simulink model "reaction_wheel_windup"  (R2021b)
settings: Solver=VariableStepAuto  StartTime=0.0  StopTime=200  RelTol=2.82e-14
values from neighbouring files (symbols this model uses):
  dt_delay = 0.01    [Reaction_wheel_new.m]
  hwdotmax = 0.004    [Reaction_wheel_new.m]    (also in test_trajectory.m)
  hwmax = 0.015    [Reaction_wheel_new.m]    (also in test_trajectory.m)
  K = 1/bode(Co*CLTF1*Go,2*pi*1)    [Reaction_wheel_new.m]
  Kd = diag([Kd1; Kd2; Kd3])    [Reaction_wheel_new.m]
  Kp = 1/bode(CLTF1*Go,2*pi*1)    [Reaction_wheel_new.m]
  p = 2*pi*100    (= 628.318530718)    [Reaction_wheel_new.m]
  qstar_BI = e2q(e,180*pi/180)    [Reaction_wheel_new.m]
  s = tf('s')    [Reaction_wheel_new.m]
  safety = 0.5    [Reaction_wheel_new.m]    (also in test_trajectory.m)
  wn = 2*pi*10    (= 62.8318530718)    [Reaction_wheel_new.m]
  z = 2*pi*0.0001    (= 0.000628318530718)    [Reaction_wheel_new.m]
  zeta = sqrt(2)/2    [Reaction_wheel_new.m]
undefined symbols (not defined in the file or in its folder): A_BP, A_PB, J_C_B, md, ms, q_PB, rcb_B, X, Y, Z
libraries: sm_lib x10, nesl_utility x4
settings Model: Creator=trisha  LastModifiedBy=trisha

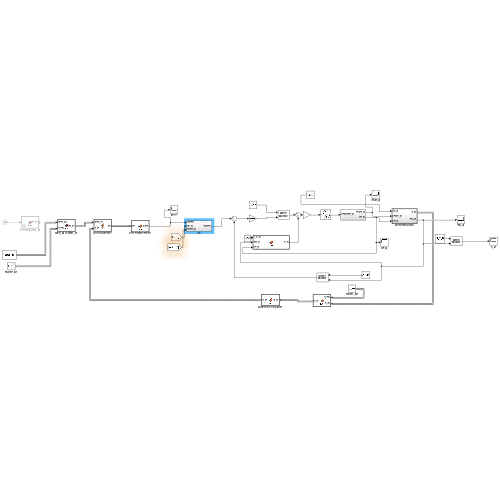
[thumbnail: Simulink's stored preview of the top-level diagram]
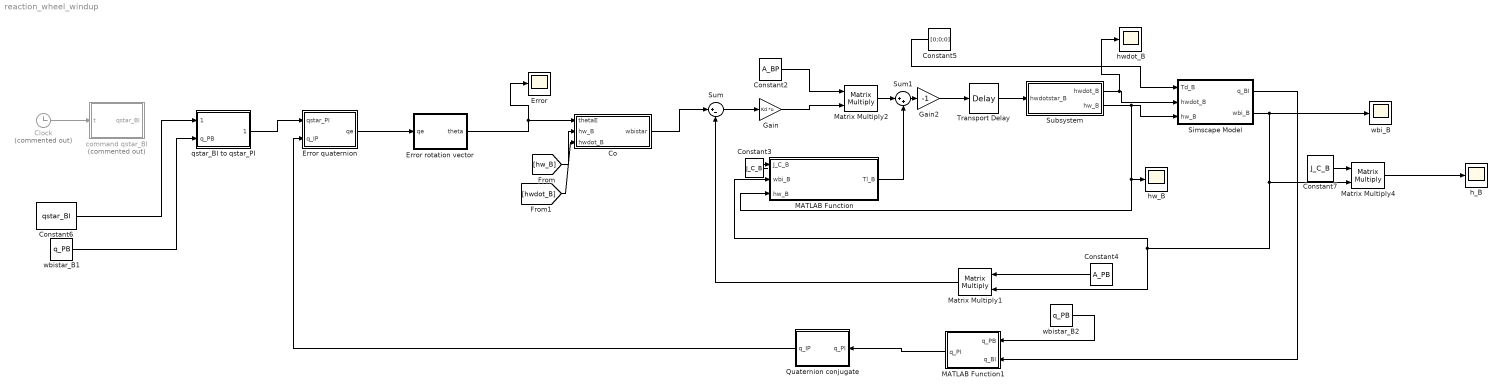
== system reaction_wheel_windup ==
  Clock : Clock  Commented=on
  Co : Subsystem
  Constant2 : Constant  Value=A_BP
  Constant3 : Constant  Value=J_C_B
  Constant4 : Constant  Value=A_PB
  Constant5 : Constant  Value=[0;0;0]
  Constant6 : Constant  Value=qstar_BI  OutDataTypeStr=Bus: qBus
  Constant7 : Constant  Value=J_C_B
  Error : Scope
  Error quaternion : MATLAB Function  TreatAsAtomicUnit=on
  "Error rotation vector " : MATLAB Function  TreatAsAtomicUnit=on
  Gain : Gain  Gain=Kd  Multiplication=Matrix(K*u) (u vector)
  Gain2 : Gain  Gain=-1
  MATLAB Function : MATLAB Function  TreatAsAtomicUnit=on
  MATLAB Function1 : MATLAB Function  TreatAsAtomicUnit=on
  Matrix Multiply1 : Product  Multiplication=Matrix(*)
  Matrix Multiply2 : Product  Multiplication=Matrix(*)
  Matrix Multiply4 : Product  Multiplication=Matrix(*)
  "Quaternion conjugate " : MATLAB Function  TreatAsAtomicUnit=on
  Simscape Model : Subsystem  TreatAsAtomicUnit=on
  Subsystem : Subsystem
  Sum : Sum  Inputs=|+-
  Sum1 : Sum  Inputs=|++
  Transport Delay : TransportDelay  DelayTime=dt_delay
  command qstar_BI : MATLAB Function  Commented=on  TreatAsAtomicUnit=on
  h_B : Scope
  hw_B : Scope
  hwdot_B : Scope
  qstar_BI to qstar_PI : MATLAB Function  TreatAsAtomicUnit=on
  wbi_B : Scope
  wbistar_B1 : Constant  Value=q_PB  VectorParams1D=off  OutDataTypeStr=Bus: qBus
  wbistar_B2 : Constant  Value=q_PB  VectorParams1D=off  OutDataTypeStr=Bus: qBus
  wires:
  Sum1/1 -> Gain2/1
  Sum/1 -> Gain/1
  Clock/1 -> command qstar_BI/1(t)
  "Quaternion conjugate "/1(q_IP) -> Error quaternion/2(q_IP)
  Constant3/1 -> MATLAB Function/1(J_C_B)
  Matrix Multiply1/1 -> Sum/2
  "Error rotation vector "/1(theta) -> Co/1(thetaE), Error/1
  Constant5/1 -> Simscape Model/1(Td_B)
  Transport Delay/1 -> Subsystem/1(hwdotstar_B)
  Constant4/1 -> Matrix Multiply1/1
  wbistar_B1/1 -> qstar_BI to qstar_PI/2(q_PB)
  Gain/1 -> Matrix Multiply2/2
  MATLAB Function/1(Tl_B) -> Sum1/2
  Error quaternion/1(qe) -> "Error rotation vector "/1(qe)
  Simscape Model/2(wbi_B) -> wbi_B/1, Matrix Multiply4/2, Matrix Multiply1/2, MATLAB Function/2(wbi_B)
  Constant2/1 -> Matrix Multiply2/1
  Simscape Model/1(q_BI) -> MATLAB Function1/2(q_BI)
  wbistar_B2/1 -> MATLAB Function1/1(q_PB)
  Co/1(wbistar) -> Sum/1
  MATLAB Function1/1(q_PI) -> "Quaternion conjugate "/1(q_PI)
  Matrix Multiply2/1 -> Sum1/1
  Gain2/1 -> Transport Delay/1
  Matrix Multiply4/1 -> h_B/1
  Constant7/1 -> Matrix Multiply4/1
  qstar_BI to qstar_PI/1(qstar_PI) -> Error quaternion/1(qstar_PI)
  Constant6/1 -> qstar_BI to qstar_PI/1(qstar_BI)
  Subsystem/2(hw_B) -> hw_B/1, MATLAB Function/3(hw_B), Simscape Model/3(hw_B)
  Subsystem/1(hwdot_B) -> hwdot_B/1, Simscape Model/2(hwdot_B)
  [hw_B] -> Co/2(hw_B)
  [hwdot_B] -> Co/3(hwdot_B)

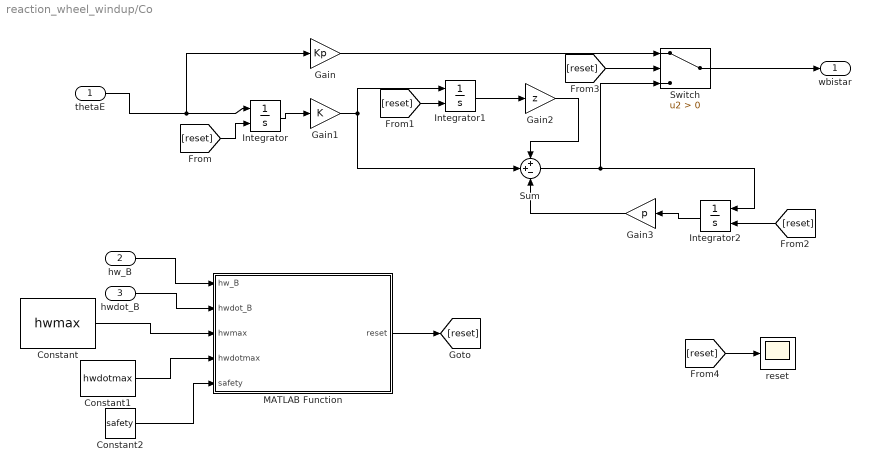
== system reaction_wheel_windup/Co ==
  thetaE : Inport
  hw_B : Inport  Port=2
  hwdot_B : Inport  Port=3
  Constant : Constant  Value=hwmax
  Constant1 : Constant  Value=hwdotmax
  Constant2 : Constant  Value=safety
  Gain : Gain  Gain=Kp
  Gain1 : Gain  Gain=K
  Gain2 : Gain  Gain=z
  Gain3 : Gain  Gain=p
  Integrator : Integrator  ExternalReset=level
  Integrator1 : Integrator  ExternalReset=level
  Integrator2 : Integrator  ExternalReset=level
  MATLAB Function : MATLAB Function  TreatAsAtomicUnit=on
  Sum : Sum  Inputs=++-
  Switch : Switch  Criteria=u2 > Threshold
  reset : Scope
  wbistar : Outport
  wires:
  Gain/1 -> Switch/1
  Switch/1 -> wbistar/1
  Integrator/1 -> Gain1/1
  Integrator1/1 -> Gain2/1
  Gain1/1 -> Sum/2, Integrator1/1
  Gain2/1 -> Sum/1
  Integrator2/1 -> Gain3/1
  Sum/1 -> Integrator2/1, Switch/3
  Gain3/1 -> Sum/3
  thetaE/1 -> Gain/1, Integrator/1
  [reset] -> Integrator/2
  [reset] -> Integrator1/2
  [reset] -> Integrator2/2
  [reset] -> Switch/2
  hw_B/1 -> MATLAB Function/1(hw_B)
  hwdot_B/1 -> MATLAB Function/2(hwdot_B)
  Constant/1 -> MATLAB Function/3(hwmax)
  Constant1/1 -> MATLAB Function/4(hwdotmax)
  Constant2/1 -> MATLAB Function/5(safety)
  MATLAB Function/1(reset) -> [reset]
  [reset] -> reset/1

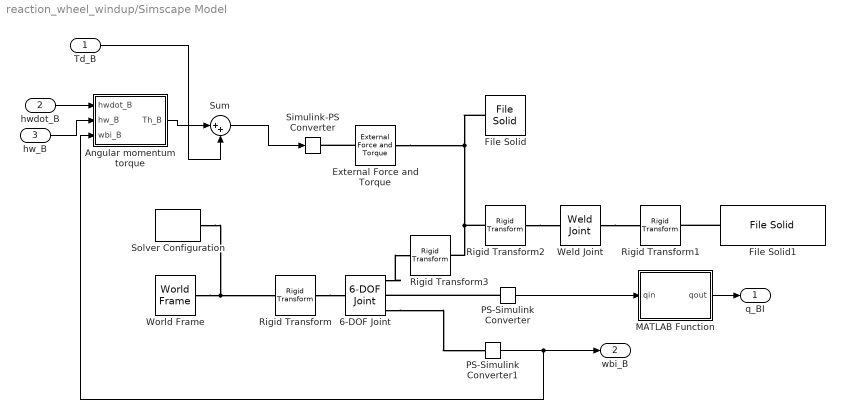
== system reaction_wheel_windup/Simscape Model ==
  Td_B : Inport
  hwdot_B : Inport  Port=2
  hw_B : Inport  Port=3
  6-DOF Joint : sm_lib/Joints/6-DOF Joint  JointMode=Normal  SenseConstraintForce=off  SenseConstraintForceX=off  SenseConstraintForceY=off  SenseConstraintForceZ=off  SenseConstraintTorque=off  SenseConstraintTorqueX=off  SenseConstraintTorqueY=off  SenseConstraintTorqueZ=off  SenseTotalForce=off  SenseTotalForceX=off  SenseTotalForceY=off  SenseTotalForceZ=off  SenseTotalTorque=off  SenseTotalTorqueX=off  SenseTotalTorqueY=off  SenseTotalTorqueZ=off  CompositeWrenchDir=FollowerOnBase  CompositeWrenchFrame=BaseFrame  PxEquilibriumPosition=0  PxEquilibriumPositionUnits=m  PxSpringStiffness=0  PxSpringStiffnessUnits=N/m  PxDampingCoefficient=0  PxDampingCoefficientUnits=N/(m/s)  PxTorqueActuationMode=NoTorque  PxMotionActuationMode=ComputedMotion  PxSensePosition=off  PxSenseVelocity=off  PxSenseAcceleration=off  PxSenseTorqueForce=off  PxSenseLowerLimitTorqueForce=off  PxSenseUpperLimitTorqueForce=off  PxLowerLimitSpecify=off  PxLowerLimitBound=-1  PxLowerLimitBoundUnits=m  PxLowerLimitStiffness=1e6  PxLowerLimitStiffnessUnits=N/m  PxLowerLimitDamping=1e3  PxLowerLimitDampingUnits=N/(m/s)  PxLowerLimitTransitionRegionWidth=1e-4  PxLowerLimitTransitionRegionWidthUnits=m  PxUpperLimitSpecify=off  PxUpperLimitBound=1  PxUpperLimitBoundUnits=m  PxUpperLimitStiffness=1e6  PxUpperLimitStiffnessUnits=N/m  PxUpperLimitDamping=1e3  PxUpperLimitDampingUnits=N/(m/s)  PxUpperLimitTransitionRegionWidth=1e-4  PxUpperLimitTransitionRegionWidthUnits=m  PxPositionTargetSpecify=off  PxPositionTargetPriority=High  PxPositionTargetValue=0  PxPositionTargetValueUnits=m  PxVelocityTargetSpecify=off  PxVelocityTargetPriority=High  PxVelocityTargetValue=0  PxVelocityTargetValueUnits=m/s  PyEquilibriumPosition=0  PyEquilibriumPositionUnits=m  PySpringStiffness=0  PySpringStiffnessUnits=N/m  PyDampingCoefficient=0  PyDampingCoefficientUnits=N/(m/s)  PyTorqueActuationMode=NoTorque  PyMotionActuationMode=ComputedMotion  PySensePosition=off  PySenseVelocity=off  PySenseAcceleration=off  PySenseTorqueForce=off  PySenseLowerLimitTorqueForce=off  PySenseUpperLimitTorqueForce=off  PyLowerLimitSpecify=off  PyLowerLimitBound=-1  PyLowerLimitBoundUnits=m  PyLowerLimitStiffness=1e6  PyLowerLimitStiffnessUnits=N/m  PyLowerLimitDamping=1e3  PyLowerLimitDampingUnits=N/(m/s)  PyLowerLimitTransitionRegionWidth=1e-4  PyLowerLimitTransitionRegionWidthUnits=m  PyUpperLimitSpecify=off  PyUpperLimitBound=1  PyUpperLimitBoundUnits=m  PyUpperLimitStiffness=1e6  PyUpperLimitStiffnessUnits=N/m  PyUpperLimitDamping=1e3  PyUpperLimitDampingUnits=N/(m/s)  PyUpperLimitTransitionRegionWidth=1e-4  PyUpperLimitTransitionRegionWidthUnits=m  PyPositionTargetSpecify=off  PyPositionTargetPriority=High  PyPositionTargetValue=0  PyPositionTargetValueUnits=m  PyVelocityTargetSpecify=off  PyVelocityTargetPriority=High  PyVelocityTargetValue=0  PyVelocityTargetValueUnits=m/s  PzEquilibriumPosition=0  PzEquilibriumPositionUnits=m  PzSpringStiffness=0  PzSpringStiffnessUnits=N/m  PzDampingCoefficient=0  PzDampingCoefficientUnits=N/(m/s)  PzTorqueActuationMode=NoTorque  PzMotionActuationMode=ComputedMotion  PzSensePosition=off  PzSenseVelocity=off  PzSenseAcceleration=off  PzSenseTorqueForce=off  PzSenseLowerLimitTorqueForce=off  PzSenseUpperLimitTorqueForce=off  PzLowerLimitSpecify=off  PzLowerLimitBound=-1  PzLowerLimitBoundUnits=m  PzLowerLimitStiffness=1e6  PzLowerLimitStiffnessUnits=N/m  PzLowerLimitDamping=1e3  PzLowerLimitDampingUnits=N/(m/s)  PzLowerLimitTransitionRegionWidth=1e-4  PzLowerLimitTransitionRegionWidthUnits=m  PzUpperLimitSpecify=off  PzUpperLimitBound=1  PzUpperLimitBoundUnits=m  PzUpperLimitStiffness=1e6  PzUpperLimitStiffnessUnits=N/m  PzUpperLimitDamping=1e3  PzUpperLimitDampingUnits=N/(m/s)  PzUpperLimitTransitionRegionWidth=1e-4  PzUpperLimitTransitionRegionWidthUnits=m  PzPositionTargetSpecify=off  PzPositionTargetPriority=High  PzPositionTargetValue=0  PzPositionTargetValueUnits=m  PzVelocityTargetSpecify=off  PzVelocityTargetPriority=High  PzVelocityTargetValue=0  PzVelocityTargetValueUnits=m/s  SphDefPosRotationMethod=None  SphDefPosRotationAngleUnits=deg  SphDefPosRotationStandardAxis=+Z  SphDefPosRotationAngle=0.0  SphDefPosRotationArbitraryAxis=[0 0 1]  SphDefPosFollAlignAxisA=+X  SphDefPosBaseAlignAxisA=+Y  SphDefPosFollAlignAxisB=+Y  SphDefPosBaseAlignAxisB=+Z  SphDefPosRotationSequenceAxes=FollowerAxes  SphDefPosRotationSequence=XYX  SphDefPosRotationSequenceAngles=[0 0 0]  SphDefPosRotationSequenceAnglesUnits=deg  SphDefPosRotationMatrix=[1 0 0; 0 1 0; 0 0 1]  SphEqPosRotationMethod=None  SphEqPosRotationAngleUnits=deg  SphEqPosRotationStandardAxis=+Z  SphEqPosRotationAngle=0.0  SphEqPosRotationArbitraryAxis=[0 0 1]  SphEqPosFollAlignAxisA=+X  SphEqPosBaseAlignAxisA=+Y  SphEqPosFollAlignAxisB=+Y  SphEqPosBaseAlignAxisB=+Z  SphEqPosRotationSequenceAxes=FollowerAxes  SphEqPosRotationSequence=XYX  SphEqPosRotationSequenceAngles=[0 0 0]  SphEqPosRotationSequenceAnglesUnits=deg  SphEqPosRotationMatrix=[1 0 0; 0 1 0; 0 0 1]  SphSpringStiffness=0  SphSpringStiffnessUnits=N*m/deg  SphDampingCoefficient=0  SphDampingCoefficientUnits=N*m/(deg/s)  SphActuateTorqueX=off  SphActuateTorqueY=off  SphActuateTorqueZ=off  SphActuateTorque=off  SphTorqueActuationMode=NoTorque  SphMotionActuationMode=ComputedMotion  SphActuationFrame=BaseFrame  SphSensePosition=on  SphSenseVelocityX=off  SphSenseVelocityY=off  SphSenseVelocityZ=off  SphSenseVelocity=on  SphSenseAccelerationX=off  SphSenseAccelerationY=off  SphSenseAccelerationZ=off  SphSenseAcceleration=off  SphSenseTorqueX=off  SphSenseTorqueY=off  SphSenseTorqueZ=off  SphSenseTorqueForce=off  SphSenseLowerLimitTorqueMag=off  SphSenseUpperLimitTorqueMag=off  SphSensingFrame=FollowerFrame  SphLowerLimitSpecify=off  SphLowerLimitBound=15  SphLowerLimitBoundUnits=deg  SphLowerLimitStiffness=1e4  SphLowerLimitStiffnessUnits=N*m/deg  SphLowerLimitDamping=10  SphLowerLimitDampingUnits=N*m/(deg/s)  SphLowerLimitTransitionRegionWidth=0.1  SphLowerLimitTransitionRegionWidthUnits=deg  SphUpperLimitSpecify=off  SphUpperLimitBound=45  SphUpperLimitBoundUnits=deg  SphUpperLimitStiffness=1e4  SphUpperLimitStiffnessUnits=N*m/deg  SphUpperLimitDamping=10  SphUpperLimitDampingUnits=N*m/(deg/s)  SphUpperLimitTransitionRegionWidth=0.1  SphUpperLimitTransitionRegionWidthUnits=deg  SphPositionTargetRotationMethod=RotationMatrix  SphPositionTargetRotationAngleUnits=deg  SphPositionTargetRotationStandardAxis=+Z  SphPositionTargetRotationAngle=0.0  SphPositionTargetRotationArbitraryAxis=[0 0 1]  SphPositionTargetFollAlignAxisA=+X  SphPositionTargetBaseAlignAxisA=+Y  SphPositionTargetFollAlignAxisB=+Y  SphPositionTargetBaseAlignAxisB=+Z  SphPositionTargetRotationSequenceAxes=FollowerAxes  SphPositionTargetRotationSequence=XYX  SphPositionTargetRotationSequenceAngles=[0 0 0]  SphPositionTargetRotationSequenceAnglesUnits=deg  SphPositionTargetRotationMatrix=A0_IB  SphPositionTargetSpecify=on  SphPositionTargetPriority=High  SphVelocityTargetValue=wbi0_B  SphVelocityTargetValueUnits=rad/s  SphVelocityTargetSpecify=on  SphVelocityTargetPriority=High  SphVelocityTargetInFollowerFrame=on
  "Angular momentum torque " : MATLAB Function  TreatAsAtomicUnit=on
  External Force and Torque : sm_lib/Forces and Torques/External Force and Torque  ForceResolutionFrame=AttachedFrame  EnableForceX=off  EnableForceY=off  EnableForceZ=off  EnableForce=off  TorqueResolutionFrame=AttachedFrame  EnableTorqueX=off  EnableTorqueY=off  EnableTorqueZ=off  EnableTorque=on
  File Solid : sm_lib/Body Elements/File Solid  ExtGeomFileName=/Users/trisha/Downloads/Structure.STL  UnitType=Custom  ExtGeomFileUnits=mm  StepReaderType=HEX  ExportConvexHullGeometry=off  InertiaType=Custom  Mass=ms  MassUnits=kg  CenterOfMass=rsb_B  CenterOfMassUnits=m  MomentsOfInertia=Ms_S_B  MomentsOfInertiaUnits=kg*m^2  ProductsOfInertia=Ps_S_B  ProductsOfInertiaUnits=kg*m^2  BasedOnType=DensityFromFile  Density=1000  DensityUnits=kg/m^3  DoExposeReferenceFrame=on  SerializedFrames=<Frames/>  GraphicType=FromGeometry  MarkerShape=Sphere  MarkerSize=10  GraphicVisPropType=SimpleVisualProperties  GraphicDiffuseColor=[0.5 0.5 0.5]  GraphicSpecularColor=[0.5 0.5 0.5 1.0]  GraphicAmbientColor=[0.15 0.15 0.15 1.0]  GraphicEmissiveColor=[0.0 0.0 0.0 1.0]  GraphicShininess=75  GraphicOpacity=1.0
  File Solid1 : sm_lib/Body Elements/File Solid  ExtGeomFileName=/Users/trisha/Downloads/Deployable.STL  UnitType=Custom  ExtGeomFileUnits=mm  StepReaderType=HEX  ExportConvexHullGeometry=off  InertiaType=Custom  Mass=md  MassUnits=kg  CenterOfMass=rdb_B  CenterOfMassUnits=m  MomentsOfInertia=Md_D_B  MomentsOfInertiaUnits=kg*m^2  ProductsOfInertia=Pd_D_B  ProductsOfInertiaUnits=kg*m^2  BasedOnType=DensityFromFile  Density=1000  DensityUnits=kg/m^3  DoExposeReferenceFrame=on  SerializedFrames=<Frames/>  GraphicType=FromGeometry  MarkerShape=Sphere  MarkerSize=10  GraphicVisPropType=SimpleVisualProperties  GraphicDiffuseColor=[0.5 0.5 0.5]  GraphicSpecularColor=[0.5 0.5 0.5 1.0]  GraphicAmbientColor=[0.15 0.15 0.15 1.0]  GraphicEmissiveColor=[0.0 0.0 0.0 1.0]  GraphicShininess=75  GraphicOpacity=1.0
  MATLAB Function : MATLAB Function  TreatAsAtomicUnit=on
  PS-Simulink Converter : nesl_utility/PS-Simulink Converter  PhysicalDomain=network_engine_domain  SubClassName=ps_output  LeftPortType=input  RightPortType=output  PseudoPeriodic=off  Frequencies=[]  Unit=inherit  AffineConversion=off
      settings: SourceProductBaseCode=PW,SS
  PS-Simulink Converter1 : nesl_utility/PS-Simulink Converter  PhysicalDomain=network_engine_domain  SubClassName=ps_output  LeftPortType=input  RightPortType=output  PseudoPeriodic=off  Frequencies=[]  Unit=inherit  AffineConversion=off
      settings: SourceProductBaseCode=PW,SS
  Rigid Transform : sm_lib/Frames and Transforms/Rigid Transform  TranslationMethod=Cartesian  TranslationStandardOffset=0  TranslationLengthUnit=m  TranslationStandardAxis=+Z  TranslationCartesianOffset=rcb_B  TranslationROffset=0  TranslationROffsetUnits=m  TranslationZOffset=0  TranslationZOffsetUnits=m  TranslationThetaOffset=0  TranslationThetaOffsetUnits=deg  RotationMethod=None  RotationAngleUnits=deg  RotationStandardAxis=+Z  RotationAngle=0.0  RotationArbitraryAxis=[0 0 1]  FollAlignAxisA=+X  BaseAlignAxisA=+Y  FollAlignAxisB=+Y  BaseAlignAxisB=+Z  RotationSequenceAxes=FollowerAxes  RotationSequence=XYX  RotationSequenceAngles=[0 0 0]  RotationSequenceAnglesUnits=deg  RotationMatrix=[1 0 0; 0 1 0; 0 0 1]
  Rigid Transform1 : sm_lib/Frames and Transforms/Rigid Transform  TranslationMethod=Cartesian  TranslationStandardOffset=0  TranslationLengthUnit=m  TranslationStandardAxis=+Z  TranslationCartesianOffset=-rcb_B  TranslationROffset=0  TranslationROffsetUnits=m  TranslationZOffset=0  TranslationZOffsetUnits=m  TranslationThetaOffset=0  TranslationThetaOffsetUnits=deg  RotationMethod=None  RotationAngleUnits=deg  RotationStandardAxis=+Z  RotationAngle=0.0  RotationArbitraryAxis=[0 0 1]  FollAlignAxisA=+X  BaseAlignAxisA=+Y  FollAlignAxisB=+Y  BaseAlignAxisB=+Z  RotationSequenceAxes=FollowerAxes  RotationSequence=XYX  RotationSequenceAngles=[0 0 0]  RotationSequenceAnglesUnits=deg  RotationMatrix=[1 0 0; 0 1 0; 0 0 1]
  Rigid Transform2 : sm_lib/Frames and Transforms/Rigid Transform  TranslationMethod=Cartesian  TranslationStandardOffset=0  TranslationLengthUnit=m  TranslationStandardAxis=+Z  TranslationCartesianOffset=rcb_B  TranslationROffset=0  TranslationROffsetUnits=m  TranslationZOffset=0  TranslationZOffsetUnits=m  TranslationThetaOffset=0  TranslationThetaOffsetUnits=deg  RotationMethod=None  RotationAngleUnits=deg  RotationStandardAxis=+Z  RotationAngle=0.0  RotationArbitraryAxis=[0 0 1]  FollAlignAxisA=+X  BaseAlignAxisA=+Y  FollAlignAxisB=+Y  BaseAlignAxisB=+Z  RotationSequenceAxes=FollowerAxes  RotationSequence=XYX  RotationSequenceAngles=[0 0 0]  RotationSequenceAnglesUnits=deg  RotationMatrix=[1 0 0; 0 1 0; 0 0 1]
  Rigid Transform3 : sm_lib/Frames and Transforms/Rigid Transform  TranslationMethod=Cartesian  TranslationStandardOffset=0  TranslationLengthUnit=m  TranslationStandardAxis=+Z  TranslationCartesianOffset=-rcb_B  TranslationROffset=0  TranslationROffsetUnits=m  TranslationZOffset=0  TranslationZOffsetUnits=m  TranslationThetaOffset=0  TranslationThetaOffsetUnits=deg  RotationMethod=None  RotationAngleUnits=deg  RotationStandardAxis=+Z  RotationAngle=0.0  RotationArbitraryAxis=[0 0 1]  FollAlignAxisA=+X  BaseAlignAxisA=+Y  FollAlignAxisB=+Y  BaseAlignAxisB=+Z  RotationSequenceAxes=FollowerAxes  RotationSequence=XYX  RotationSequenceAngles=[0 0 0]  RotationSequenceAnglesUnits=deg  RotationMatrix=[1 0 0; 0 1 0; 0 0 1]
  Simulink-PS Converter : nesl_utility/Simulink-PS Converter  PhysicalDomain=network_engine_domain  SubClassName=ps_input  LeftPortType=input  RightPortType=output  PseudoPeriodic=off  Frequencies=[]  NoiseDistribution=none  NoiseParameters=[]  Unit=1  AffineConversion=off  FilteringAndDerivatives=provide  SimscapeFilterOrder=1  InputFilterTimeConstant=0.001  UdotUserProvided=0
      settings: SourceProductBaseCode=PW,SS
  Solver Configuration : nesl_utility/Solver Configuration  PhysicalDomain=network_engine_domain  SubClassName=solver  LeftPortType=input  RightPortType=generic  Tones=[]  Harmonics=[]  SimulateNoise=off  Profile=off  UseLocalSampling=off  EnableSwitchedLinearOptims=on  FrequencyDomain=off  UseCCode=off  RelTol=0.001  AbsTol=1e-06  MinStep=1e-09  ToWorkspace=off  RevertToSquareIcSolve=off  NumHomotopyIterations=100  PhasorMode=off  PhasorModeNumHarmonics=1  DoDC=off  ResidualTolerance=1e-09  UseLocalSolver=off  LocalSolverChoice=NE_BACKWARD_EULER_ADVANCER  LocalSolverSampleTime=0.001  DoFixedCost=off  MaxNonlinIter=3  MaxModeIter=2  ComputeImpulses=off  ImpulseIterations=2  LinearAlgebra=auto  EquationFormulation=NE_TIME_EF  DelaysMemoryBudget=1024  AutomaticFiltering=on  FilteringTimeConstant=0.001  PartitionStorageMethod=AS_NEEDED  PartitionMemoryBudget=1024  PartitionMethod=ROBUST
      settings: SourceProductBaseCode=PW,SS
  Sum : Sum  Inputs=|++
  Weld Joint : sm_lib/Joints/Weld Joint  JointMode=Normal  SenseConstraintForce=off  SenseConstraintForceX=off  SenseConstraintForceY=off  SenseConstraintForceZ=off  SenseConstraintTorque=off  SenseConstraintTorqueX=off  SenseConstraintTorqueY=off  SenseConstraintTorqueZ=off  SenseTotalForce=off  SenseTotalForceX=off  SenseTotalForceY=off  SenseTotalForceZ=off  SenseTotalTorque=off  SenseTotalTorqueX=off  SenseTotalTorqueY=off  SenseTotalTorqueZ=off  CompositeWrenchDir=FollowerOnBase  CompositeWrenchFrame=BaseFrame
  World Frame : sm_lib/Frames and Transforms/World Frame
  q_BI : Outport  OutDataTypeStr=Bus: qBus
  wbi_B : Outport  Port=2
  wires:
  PS-Simulink Converter/1 -> MATLAB Function/1(qin)
  MATLAB Function/1(qout) -> q_BI/1
  PS-Simulink Converter1/1 -> "Angular momentum torque "/3(wbi_B), wbi_B/1
  Td_B/1 -> Sum/2
  "Angular momentum torque "/1(Th_B) -> Sum/1
  Sum/1 -> Simulink-PS Converter/1
  hwdot_B/1 -> "Angular momentum torque "/1(hwdot_B)
  hw_B/1 -> "Angular momentum torque "/2(hw_B)
  connections:
  Rigid Transform/RConn1 -- 6-DOF Joint/LConn1
  World Frame/RConn1 -- Rigid Transform/LConn1 -- Solver Configuration/RConn1
  Rigid Transform2/RConn1 -- Weld Joint/LConn1
  Weld Joint/RConn1 -- Rigid Transform1/LConn1
  File Solid1/RConn1 -- Rigid Transform1/RConn1
  File Solid/RConn1 -- Rigid Transform2/LConn1 -- Rigid Transform3/RConn1 -- External Force and Torque/RConn1
  External Force and Torque/LConn1 -- Simulink-PS Converter/RConn1
  PS-Simulink Converter/LConn1 -- 6-DOF Joint/RConn2
  6-DOF Joint/RConn3 -- PS-Simulink Converter1/LConn1
  6-DOF Joint/RConn1 -- Rigid Transform3/LConn1

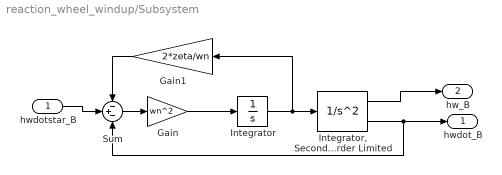
== system reaction_wheel_windup/Subsystem ==
  hwdotstar_B : Inport
  Gain : Gain  Gain=wn^2
  Gain1 : Gain  Gain=2*zeta/wn
  Integrator : Integrator
  "Integrator, Second-Order Limited" : SecondOrderIntegrator  ICX=hw0_B  LimitX=on  UpperLimitX=hwmax  LowerLimitX=-hwmax  LimitDXDT=on  UpperLimitDXDT=hwdotmax  LowerLimitDXDT=-hwdotmax
  Sum : Sum  Inputs=-+-
  hwdot_B : Outport
  hw_B : Outport  Port=2
  wires:
  Integrator/1 -> Gain1/1, "Integrator, Second-Order Limited"/1
  Gain/1 -> Integrator/1
  Sum/1 -> Gain/1
  hwdotstar_B/1 -> Sum/2
  "Integrator, Second-Order Limited"/1 -> hw_B/1
  "Integrator, Second-Order Limited"/2 -> Sum/3, hwdot_B/1
  Gain1/1 -> Sum/1

== matlab function reaction_wheel_windup/MATLAB Function ==
  data: J_C_B input; Tl_B output; wbi_B input; hw_B input
function Tl_B = fcn(J_C_B,wbi_B,hw_B)

Tl_B = cross(wbi_B,J_C_B*wbi_B+hw_B);

== matlab function reaction_wheel_windup/command qstar_BI ==
  data: qstar_BI output Bus: qBus; t input
function qstar_BI = fcn(t)
  e = [1;0;0];
  e = e/norm(e);
%   angle = 2*pi*t*0.1 ;
 
  angle = 180*pi/180;
%   angle = 0 ;
  
%   angle = pi; 
  qstar_BI = e2q(e,angle);

== matlab function reaction_wheel_windup/qstar_BI to qstar_PI ==
  data: qstar_BI input Bus: qBus; qstar_PI output Bus: qBus; q_PB input Bus: qBus
function qstar_PI = fcn(qstar_BI,q_PB)

qstar_PI = qX(qstar_BI,q_PB);

== matlab function reaction_wheel_windup/Simscape Model/MATLAB Function ==
  data: qin input; qout output Bus: qBus
function qout = fcn(qin)
qout.s = qin(1);
qout.v = qin(2:4);

== matlab function reaction_wheel_windup/Error quaternion ==
  data: qstar_PI input Bus: qBus; qe output Bus: qBus; q_IP input Bus: qBus
function qe = fcn(qstar_PI,q_IP)

qe = qX(qstar_PI,q_IP);

== matlab function reaction_wheel_windup/Error rotation vector  ==
  data: qe input Bus: qBus; theta output
function theta = fcn(qe)

qe = qUnit(qe);
[e, angle] = q2e(qe);
theta = e*angle;

== matlab function reaction_wheel_windup/MATLAB Function1 ==
  data: q_PB input Bus: qBus; q_PI output Bus: qBus; q_BI input Bus: qBus
function q_PI = fcn(q_PB,q_BI)

q_PI = qX(q_PB,q_BI);

== matlab function reaction_wheel_windup/Quaternion conjugate  ==
  data: q_PI input Bus: qBus; q_IP output Bus: qBus
function q_IP = fcn(q_PI)
q_IP = qT(q_PI);

== matlab function reaction_wheel_windup/Co/MATLAB Function ==
  data: hw_B input; reset output; hwdot_B input; hwmax input; hwdotmax input; safety input
function reset = fcn(hw_B, hwdot_B, hwmax, hwdotmax,safety)

reset = 0;

if max(abs(hw_B)) >= hwmax*safety || max(abs(hwdot_B)) >= hwdotmax*safety
    reset = 1;
end

== matlab function reaction_wheel_windup/Simscape Model/Angular momentum torque  ==
  data: hwdot_B input; Th_B output; hw_B input; wbi_B input
function Th_B = fcn(hwdot_B,hw_B,wbi_B)

Th_B = -hwdot_B - cross(wbi_B,hw_B);
